simulink model "Copy_of_Clark"  (R2022b)
settings: Solver=ode4  StartTime=0.0  StopTime=1  FixedStep=1e-5  RelTol=1e-3
values from neighbouring files (symbols this model uses):
  E = 700    [FOCinit.m]
  f = 0.005    [FOCinit.m]
  J = 0.006    [FOCinit.m]
  Kie = 3 / (t5e * Ke)    (= 216000)    [FOCinit.m]
  Kif = 3 / (t5f * Kf)    (= 254.237288136)    [FOCinit.m]
  Kim = 3 / (t5m * Km)    (= 0.03)    [FOCinit.m]
  Kpe = taue * Kie    (= 2830.4)    [FOCinit.m]
  Kpf = tauf * Kif    (= 14.1242937853)    [FOCinit.m]
  Kpm = taum * Kim    (= 0.036)    [FOCinit.m]
  Lr = 0.075    [FOCinit.m]
  Ls = 0.280    (= 0.28)    [FOCinit.m]
  Msr = 0.118    [FOCinit.m]
  P = 2    [FOCinit.m]
  Poff = [1 1 1 1 1 1 1 1 1 1 1 1 1 1 1 1 1 1 ; 1 0 0 1 1 0 0 1 0 0 1 1 0 0 1 1 0 1; 1 1 0 0 1 0 0 1 1 0 0 1 1 0 1 1 0 0]'    [FOCinit.m]
  Rr = 1.35    [FOCinit.m]
  Rs = 7.2    [FOCinit.m]
  Ts = 1/fs    (= 0.0001)    [FOCinit.m]
libraries: slpidlib x4, simulink_extras x4, simulink x2, mcbcontrolslib x2
settings Model: Creator=ZinouAb  LastModifiedBy=ZinouAb
settings DebuggingCC: ParameterOverflowMsg=none  ParameterUnderflowMsg=error

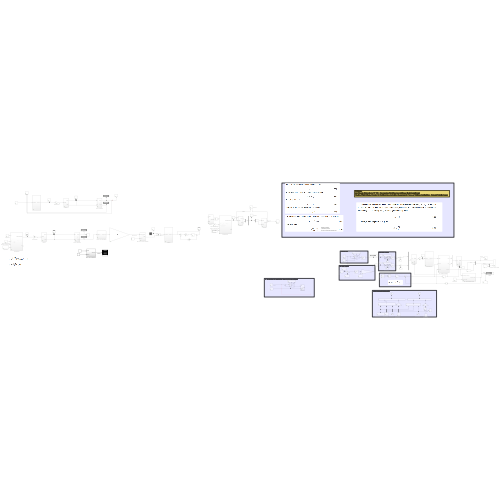
[thumbnail: Simulink's stored preview of the top-level diagram]
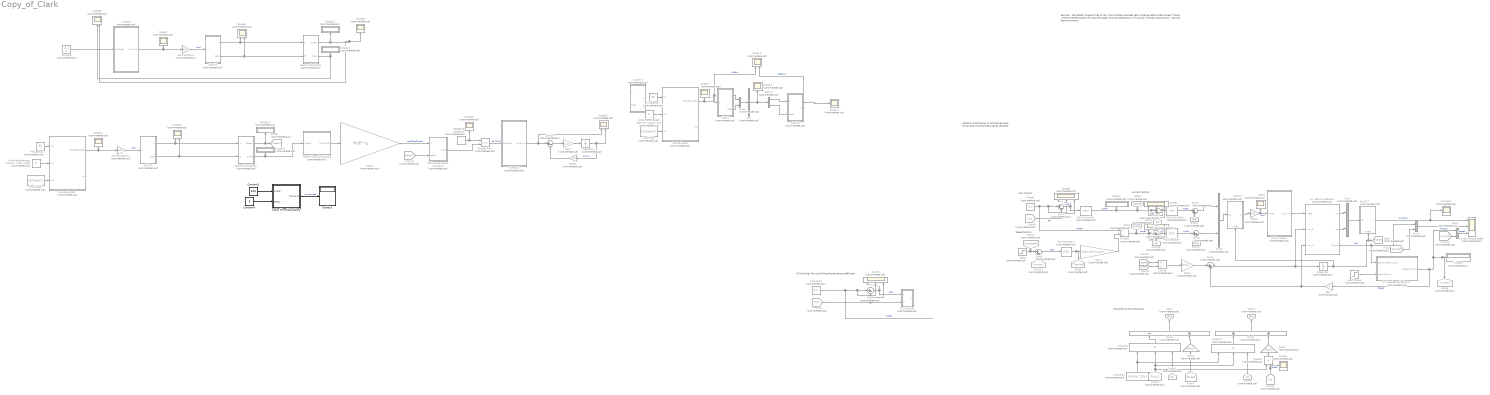
== system Copy_of_Clark ==
  note: Current Control
  note: Disturbance Compensation
  note: Notation Américaine:
      | p: Nombre de poles et
      | non pas le nombre des paires de poles
  note: Speed Control
  note: Sources :
      | Lab Sheets (Supports de TP UE - Commandes évoluées des systèmes électrotechniques)
      | Thesis : Field-Oriented Control for Squirrel-Cage Induction Generators in Pump as Turbines Applications - Samuel Ferreira Amaro
  note: Flux Control
  note: IP Controller (for controlling the damping coefficient)
  Alpha leDéphasage entre les courants (rad) : Constant  Commented=on  Value=0
  Alpha leDéphasage entre les courants (rad)1 : Constant  Commented=on  Value=0
  Amplitude : Constant  Commented=on  Value=220*sqrt(2)
  Amplitude1 : Constant  Commented=on  Value=220*sqrt(2)
  ClarkT : Subsystem  Commented=on
  ClarkT-1 : Subsystem  Commented=on
  ClarkT-2 : Subsystem  Commented=on
  ClarkT1 : Subsystem  Commented=on
  ClarkT2 : Subsystem  Commented=on
  Constant : Constant  Commented=on  Value=[1 1 0]
  Constant1 : Constant  Commented=on  Value=(Ls-(Msr^2)/Lr)
  Constant2 : Constant  Commented=on  Value=0.5
  Constant3 : Constant  Value=140
  Constant4 : Constant  Value=3
  CosineWaves : Subsystem  Commented=on
  CosineWaves1 : Subsystem  Commented=on
  Current,Torque,Speed : Scope  Commented=on  NumInputPorts=3
  Currents : Scope  Commented=on
  Demux : Demux  Commented=on  Outputs=2
  Display{,1..4} (5 alike) : Display  Commented=on
  Display5 : Display
  Divide : Product  Commented=on  Inputs=*/
  Divide1 : Product  Commented=on  Inputs=/*
  Frdref1 : Constant  Commented=on  Value=0.5
  From : From  Commented=on  GotoTag=Temref
  From1 : From  Commented=on  GotoTag=Isd  TagVisibility=global
  From10 : From  Commented=on  GotoTag=Frd  TagVisibility=global
  From11 : From  Commented=on  GotoTag=Isdref
  From12 : From  Commented=on  GotoTag=Isqref
  From13 : From  Commented=on  GotoTag=wmec
  From14 : From  Commented=on  GotoTag=wmecref
  From15 : From  Commented=on  GotoTag=Isq  TagVisibility=global
  From16 : From  Commented=on  GotoTag=Sector
  From2 : From  Commented=on  GotoTag=Ed
  From3 : From  Commented=on  GotoTag=Eq
  From4 : From  Commented=on  GotoTag=Puls_S  TagVisibility=global
  From5 : From  Commented=on  GotoTag=Isq  TagVisibility=global
  From6 : From  Commented=on  GotoTag=Frd  TagVisibility=global
  From7 : From  Commented=on  GotoTag=dFrddt  TagVisibility=global
  From8 : From  Commented=on  GotoTag=Isd  TagVisibility=global
  From9 : From  Commented=on  GotoTag=Frd  TagVisibility=global
  Fréquence : Constant  Commented=on  Value=50
  Fréquence1 : Constant  Commented=on  Value=50
  Gain : Gain  Commented=on  Gain=P
  Gain1 : Gain  Commented=on  Gain=(2/3)*(1/P)*(Lr/Msr)
  Gain2 : Gain  Commented=on  Gain=1/E
  Gain3 : Gain  Commented=on  Gain=Rr/Lr
  Gain4 : Gain  Commented=on  Gain=Msr/Lr
  Gain5 : Gain  Commented=on  Gain=Msr/Lr
  Gain6 : Gain  Commented=on  Gain=Poff  Multiplication=Matrix(K*u)
  Gain7 : Gain  Commented=on  Gain=1/Ls
  Gain8 : Gain  Commented=on  Gain=22
  Goto : Goto  Commented=on  GotoTag=Ed
  Goto1 : Goto  Commented=on  GotoTag=Eq
  Goto2 : Goto  Commented=on  GotoTag=Temref
  Goto3 : Goto  Commented=on  GotoTag=Isdref
  Goto4 : Goto  Commented=on  GotoTag=Isqref
  Goto5 : Goto  Commented=on  GotoTag=wmec
  Goto6 : Goto  Commented=on  GotoTag=wmecref
  Goto7 : Goto  Commented=on  GotoTag=thetas  TagVisibility=global
  Goto8 : Goto  Commented=on  GotoTag=Sector
  GreaterThan : RelationalOperator  Commented=on  OutDataTypeStr=boolean  RndMeth=Simplest  InputSameDT=off
  IM - Electric Behavior : Subsystem  Commented=on
  IM - Mechanical Behavior : Subsystem  Commented=on
  IP Controller : Subsystem  Commented=on
  Integrator : Integrator  Commented=on
  Integrator1 : Integrator  Commented=on
  Inverter : Subsystem  Commented=on
  Inverter1 : Subsystem  Commented=on
  Load Torque : Step  Commented=on  Time=2  After=0.5  SampleTime=0
  Mux : Mux  Commented=on  Inputs=1
  Mux{1..5} (5 alike) : Mux  Commented=on  Inputs=2
  "Normalization " : Gain  Commented=on  Gain=1/E
  Normalization 1 : Gain  Commented=on  Gain=1/E
  Off time per sector calculator : Subsystem  Commented=on
  PID Controller : slpidlib/PID Controller  Commented=on  Controller=PI  Form=Parallel  TimeDomain=Continuous-time  UseExternalTs=off  SampleTime=-1  IntegratorMethod=Forward Euler  FilterMethod=Forward Euler  ControllerParametersSource=internal  P=Kpe  I=Kie  UseKiTs=off  D=0  N=100  UseFilter=on  TunerSelectOption=Transfer Function Based (PID Tuner App)  InitialConditionSource=internal  InitialConditionForIntegrator=0  InitialConditionForFilter=0  DifferentiatorICPrevScaledInput=0  ExternalReset=none  TrackingMode=off  Kt=1  LimitOutput=off  SatLimitsSource=internal  UpperSaturationLimit=inf  LowerSaturationLimit=-inf  LinearizeAsGain=on  AntiWindupMode=none  Kb=1  LimitIntegrator=off  UpperIntegratorSaturationLimit=inf  LowerIntegratorSaturationLimit=-inf  POutMin=[]  POutMax=[]  IOutMin=[]  IOutMax=[]  DOutMin=[]  DOutMax=[]  NOutMin=[]  NOutMax=[]  SumOutMin=[]  SumOutMax=[]  SaturationOutMin=[]  SaturationOutMax=[]  PParamMin=[]  PParamMax=[]  IParamMin=[]  IParamMax=[]  DParamMin=[]  DParamMax=[]  NParamMin=[]  NParamMax=[]  KbParamMin=[]  KbParamMax=[]  KtParamMin=[]  KtParamMax=[]  KbOutMin=[]  KbOutMax=[]  KtOutMin=[]  KtOutMax=[]  IntegratorOutMin=[]  IntegratorOutMax=[]  FilterOutMin=[]  FilterOutMax=[]  SumI1OutMin=[]  SumI1OutMax=[]  SumI2OutMin=[]  SumI2OutMax=[]  SumI3OutMin=[]  SumI3OutMax=[]  SumI4OutMin=[]  SumI4OutMax=[]  SumDOutMin=[]  SumDOutMax=[]  DifferentiatorOutMin=[]  DifferentiatorOutMax=[]  FilterDiffOutCoefMin=[]  FilterDiffOutCoefMax=[]  ReciprocalOutMin=[]  ReciprocalOutMax=[]  SumDenOutMin=[]  SumDenOutMax=[]  SumNumOutMin=[]  SumNumOutMax=[]  DivideOutMin=[]  DivideOutMax=[]  UdiffTsProdOutMin=[]  UdiffTsProdOutMax=[]  NTsProdOutMin=[]  NTsProdOutMax=[]  UintegralTsProdOutMin=[]  UintegralTsProdOutMax=[]  UngainTsProdOutMin=[]  UngainTsProdOutMax=[]  ClampingZeroOutDataTypeStr=Inherit: Inherit via back propagation  ClampingZeroOutMin=[]  ClampingZeroOutMax=[]  FilterDenConstantOutDataTypeStr=Inherit: Inherit via back propagation  FilterDenConstantOutMin=[]  FilterDenConstantOutMax=[]  PCopyOutDataTypeStr=Inherit: Inherit via back propagation  PCopyOutMin=[]  PCopyOutMax=[]  NCopyOutDataTypeStr=Inherit: Inherit via back propagation  NCopyOutMin=[]  NCopyOutMax=[]  IntegratorContinuousStateAttributes=''  IntegratorStateMustResolveToSignalObject=off  IntegratorRTWStateStorageClass=Auto  FilterContinuousStateAttributes=''  FilterStateMustResolveToSignalObject=off  FilterRTWStateStorageClass=Auto  ParallelPVariant=InternalParameters  IdealPVariant=Disabled  IVariant=InternalParameters  DVariant=Disabled  IntegratorVariant=Continuous  SatVariant=Disabled  AWVariant=Passthrough  PCopyVariant=Disabled  TRVariant=Disabled  FdbkBlocksVariant=Forward  IdealPFdbkVariant=Disabled  SatFdbkVariant=Disabled  DerivativeFilterVariant=Disabled  NVariant=Disabled  NCopyVariant=Disabled_SignalSpec  FilterICVariant=Disabled  IntegratorICVariant=InternalICs  ExternalResetVariant=Disabled  TRSumVariant=Passthrough  SumFdbkVariant=Disabled  SumVariant=Sum_PI  TsampFilterVariant=InternalTs  TsampNgainVariant=Passthrough  TsampIntegralVariant=Passthrough  ExternalSaturationOutDataTypeStr=Inherit: Same as second input
  PID Controller1 : slpidlib/PID Controller  Commented=on  Controller=PI  Form=Parallel  TimeDomain=Continuous-time  UseExternalTs=off  SampleTime=-1  IntegratorMethod=Forward Euler  FilterMethod=Forward Euler  ControllerParametersSource=internal  P=Kpe  I=Kie  UseKiTs=off  D=0  N=100  UseFilter=on  TunerSelectOption=Transfer Function Based (PID Tuner App)  InitialConditionSource=internal  InitialConditionForIntegrator=0  InitialConditionForFilter=0  DifferentiatorICPrevScaledInput=0  ExternalReset=none  TrackingMode=off  Kt=1  LimitOutput=off  SatLimitsSource=internal  UpperSaturationLimit=inf  LowerSaturationLimit=-inf  LinearizeAsGain=on  AntiWindupMode=none  Kb=1  LimitIntegrator=off  UpperIntegratorSaturationLimit=inf  LowerIntegratorSaturationLimit=-inf  POutMin=[]  POutMax=[]  IOutMin=[]  IOutMax=[]  DOutMin=[]  DOutMax=[]  NOutMin=[]  NOutMax=[]  SumOutMin=[]  SumOutMax=[]  SaturationOutMin=[]  SaturationOutMax=[]  PParamMin=[]  PParamMax=[]  IParamMin=[]  IParamMax=[]  DParamMin=[]  DParamMax=[]  NParamMin=[]  NParamMax=[]  KbParamMin=[]  KbParamMax=[]  KtParamMin=[]  KtParamMax=[]  KbOutMin=[]  KbOutMax=[]  KtOutMin=[]  KtOutMax=[]  IntegratorOutMin=[]  IntegratorOutMax=[]  FilterOutMin=[]  FilterOutMax=[]  SumI1OutMin=[]  SumI1OutMax=[]  SumI2OutMin=[]  SumI2OutMax=[]  SumI3OutMin=[]  SumI3OutMax=[]  SumI4OutMin=[]  SumI4OutMax=[]  SumDOutMin=[]  SumDOutMax=[]  DifferentiatorOutMin=[]  DifferentiatorOutMax=[]  FilterDiffOutCoefMin=[]  FilterDiffOutCoefMax=[]  ReciprocalOutMin=[]  ReciprocalOutMax=[]  SumDenOutMin=[]  SumDenOutMax=[]  SumNumOutMin=[]  SumNumOutMax=[]  DivideOutMin=[]  DivideOutMax=[]  UdiffTsProdOutMin=[]  UdiffTsProdOutMax=[]  NTsProdOutMin=[]  NTsProdOutMax=[]  UintegralTsProdOutMin=[]  UintegralTsProdOutMax=[]  UngainTsProdOutMin=[]  UngainTsProdOutMax=[]  ClampingZeroOutDataTypeStr=Inherit: Inherit via back propagation  ClampingZeroOutMin=[]  ClampingZeroOutMax=[]  FilterDenConstantOutDataTypeStr=Inherit: Inherit via back propagation  FilterDenConstantOutMin=[]  FilterDenConstantOutMax=[]  PCopyOutDataTypeStr=Inherit: Inherit via back propagation  PCopyOutMin=[]  PCopyOutMax=[]  NCopyOutDataTypeStr=Inherit: Inherit via back propagation  NCopyOutMin=[]  NCopyOutMax=[]  IntegratorContinuousStateAttributes=''  IntegratorStateMustResolveToSignalObject=off  IntegratorRTWStateStorageClass=Auto  FilterContinuousStateAttributes=''  FilterStateMustResolveToSignalObject=off  FilterRTWStateStorageClass=Auto  ParallelPVariant=InternalParameters  IdealPVariant=Disabled  IVariant=InternalParameters  DVariant=Disabled  IntegratorVariant=Continuous  SatVariant=Disabled  AWVariant=Passthrough  PCopyVariant=Disabled  TRVariant=Disabled  FdbkBlocksVariant=Forward  IdealPFdbkVariant=Disabled  SatFdbkVariant=Disabled  DerivativeFilterVariant=Disabled  NVariant=Disabled  NCopyVariant=Disabled_SignalSpec  FilterICVariant=Disabled  IntegratorICVariant=InternalICs  ExternalResetVariant=Disabled  TRSumVariant=Passthrough  SumFdbkVariant=Disabled  SumVariant=Sum_PI  TsampFilterVariant=InternalTs  TsampNgainVariant=Passthrough  TsampIntegralVariant=Passthrough  ExternalSaturationOutDataTypeStr=Inherit: Same as second input
  PID Controller2 : slpidlib/PID Controller  Commented=on  Controller=PI  Form=Parallel  TimeDomain=Continuous-time  UseExternalTs=off  SampleTime=-1  IntegratorMethod=Forward Euler  FilterMethod=Forward Euler  ControllerParametersSource=internal  P=Kpf  I=Kif  UseKiTs=off  D=0  N=100  UseFilter=on  TunerSelectOption=Transfer Function Based (PID Tuner App)  InitialConditionSource=internal  InitialConditionForIntegrator=0  InitialConditionForFilter=0  DifferentiatorICPrevScaledInput=0  ExternalReset=none  TrackingMode=off  Kt=1  LimitOutput=off  SatLimitsSource=internal  UpperSaturationLimit=inf  LowerSaturationLimit=-inf  LinearizeAsGain=on  AntiWindupMode=none  Kb=1  LimitIntegrator=off  UpperIntegratorSaturationLimit=inf  LowerIntegratorSaturationLimit=-inf  POutMin=[]  POutMax=[]  IOutMin=[]  IOutMax=[]  DOutMin=[]  DOutMax=[]  NOutMin=[]  NOutMax=[]  SumOutMin=[]  SumOutMax=[]  SaturationOutMin=[]  SaturationOutMax=[]  PParamMin=[]  PParamMax=[]  IParamMin=[]  IParamMax=[]  DParamMin=[]  DParamMax=[]  NParamMin=[]  NParamMax=[]  KbParamMin=[]  KbParamMax=[]  KtParamMin=[]  KtParamMax=[]  KbOutMin=[]  KbOutMax=[]  KtOutMin=[]  KtOutMax=[]  IntegratorOutMin=[]  IntegratorOutMax=[]  FilterOutMin=[]  FilterOutMax=[]  SumI1OutMin=[]  SumI1OutMax=[]  SumI2OutMin=[]  SumI2OutMax=[]  SumI3OutMin=[]  SumI3OutMax=[]  SumI4OutMin=[]  SumI4OutMax=[]  SumDOutMin=[]  SumDOutMax=[]  DifferentiatorOutMin=[]  DifferentiatorOutMax=[]  FilterDiffOutCoefMin=[]  FilterDiffOutCoefMax=[]  ReciprocalOutMin=[]  ReciprocalOutMax=[]  SumDenOutMin=[]  SumDenOutMax=[]  SumNumOutMin=[]  SumNumOutMax=[]  DivideOutMin=[]  DivideOutMax=[]  UdiffTsProdOutMin=[]  UdiffTsProdOutMax=[]  NTsProdOutMin=[]  NTsProdOutMax=[]  UintegralTsProdOutMin=[]  UintegralTsProdOutMax=[]  UngainTsProdOutMin=[]  UngainTsProdOutMax=[]  ClampingZeroOutDataTypeStr=Inherit: Inherit via back propagation  ClampingZeroOutMin=[]  ClampingZeroOutMax=[]  FilterDenConstantOutDataTypeStr=Inherit: Inherit via back propagation  FilterDenConstantOutMin=[]  FilterDenConstantOutMax=[]  PCopyOutDataTypeStr=Inherit: Inherit via back propagation  PCopyOutMin=[]  PCopyOutMax=[]  NCopyOutDataTypeStr=Inherit: Inherit via back propagation  NCopyOutMin=[]  NCopyOutMax=[]  IntegratorContinuousStateAttributes=''  IntegratorStateMustResolveToSignalObject=off  IntegratorRTWStateStorageClass=Auto  FilterContinuousStateAttributes=''  FilterStateMustResolveToSignalObject=off  FilterRTWStateStorageClass=Auto  ParallelPVariant=InternalParameters  IdealPVariant=Disabled  IVariant=InternalParameters  DVariant=Disabled  IntegratorVariant=Continuous  SatVariant=Disabled  AWVariant=Passthrough  PCopyVariant=Disabled  TRVariant=Disabled  FdbkBlocksVariant=Forward  IdealPFdbkVariant=Disabled  SatFdbkVariant=Disabled  DerivativeFilterVariant=Disabled  NVariant=Disabled  NCopyVariant=Disabled_SignalSpec  FilterICVariant=Disabled  IntegratorICVariant=InternalICs  ExternalResetVariant=Disabled  TRSumVariant=Passthrough  SumFdbkVariant=Disabled  SumVariant=Sum_PI  TsampFilterVariant=InternalTs  TsampNgainVariant=Passthrough  TsampIntegralVariant=Passthrough  ExternalSaturationOutDataTypeStr=Inherit: Same as second input
  PID Controller3 : slpidlib/PID Controller  Commented=on  Controller=PI  Form=Parallel  TimeDomain=Continuous-time  UseExternalTs=off  SampleTime=-1  IntegratorMethod=Forward Euler  FilterMethod=Forward Euler  ControllerParametersSource=internal  P=Kpm  I=Kim  UseKiTs=off  D=0  N=100  UseFilter=on  TunerSelectOption=Transfer Function Based (PID Tuner App)  InitialConditionSource=internal  InitialConditionForIntegrator=0  InitialConditionForFilter=0  DifferentiatorICPrevScaledInput=0  ExternalReset=none  TrackingMode=off  Kt=1  LimitOutput=off  SatLimitsSource=internal  UpperSaturationLimit=inf  LowerSaturationLimit=-inf  LinearizeAsGain=on  AntiWindupMode=none  Kb=1  LimitIntegrator=off  UpperIntegratorSaturationLimit=inf  LowerIntegratorSaturationLimit=-inf  POutMin=[]  POutMax=[]  IOutMin=[]  IOutMax=[]  DOutMin=[]  DOutMax=[]  NOutMin=[]  NOutMax=[]  SumOutMin=[]  SumOutMax=[]  SaturationOutMin=[]  SaturationOutMax=[]  PParamMin=[]  PParamMax=[]  IParamMin=[]  IParamMax=[]  DParamMin=[]  DParamMax=[]  NParamMin=[]  NParamMax=[]  KbParamMin=[]  KbParamMax=[]  KtParamMin=[]  KtParamMax=[]  KbOutMin=[]  KbOutMax=[]  KtOutMin=[]  KtOutMax=[]  IntegratorOutMin=[]  IntegratorOutMax=[]  FilterOutMin=[]  FilterOutMax=[]  SumI1OutMin=[]  SumI1OutMax=[]  SumI2OutMin=[]  SumI2OutMax=[]  SumI3OutMin=[]  SumI3OutMax=[]  SumI4OutMin=[]  SumI4OutMax=[]  SumDOutMin=[]  SumDOutMax=[]  DifferentiatorOutMin=[]  DifferentiatorOutMax=[]  FilterDiffOutCoefMin=[]  FilterDiffOutCoefMax=[]  ReciprocalOutMin=[]  ReciprocalOutMax=[]  SumDenOutMin=[]  SumDenOutMax=[]  SumNumOutMin=[]  SumNumOutMax=[]  DivideOutMin=[]  DivideOutMax=[]  UdiffTsProdOutMin=[]  UdiffTsProdOutMax=[]  NTsProdOutMin=[]  NTsProdOutMax=[]  UintegralTsProdOutMin=[]  UintegralTsProdOutMax=[]  UngainTsProdOutMin=[]  UngainTsProdOutMax=[]  ClampingZeroOutDataTypeStr=Inherit: Inherit via back propagation  ClampingZeroOutMin=[]  ClampingZeroOutMax=[]  FilterDenConstantOutDataTypeStr=Inherit: Inherit via back propagation  FilterDenConstantOutMin=[]  FilterDenConstantOutMax=[]  PCopyOutDataTypeStr=Inherit: Inherit via back propagation  PCopyOutMin=[]  PCopyOutMax=[]  NCopyOutDataTypeStr=Inherit: Inherit via back propagation  NCopyOutMin=[]  NCopyOutMax=[]  IntegratorContinuousStateAttributes=''  IntegratorStateMustResolveToSignalObject=off  IntegratorRTWStateStorageClass=Auto  FilterContinuousStateAttributes=''  FilterStateMustResolveToSignalObject=off  FilterRTWStateStorageClass=Auto  ParallelPVariant=InternalParameters  IdealPVariant=Disabled  IVariant=InternalParameters  DVariant=Disabled  IntegratorVariant=Continuous  SatVariant=Disabled  AWVariant=Passthrough  PCopyVariant=Disabled  TRVariant=Disabled  FdbkBlocksVariant=Forward  IdealPFdbkVariant=Disabled  SatFdbkVariant=Disabled  DerivativeFilterVariant=Disabled  NVariant=Disabled  NCopyVariant=Disabled_SignalSpec  FilterICVariant=Disabled  IntegratorICVariant=InternalICs  ExternalResetVariant=Disabled  TRSumVariant=Passthrough  SumFdbkVariant=Disabled  SumVariant=Sum_PI  TsampFilterVariant=InternalTs  TsampNgainVariant=Passthrough  TsampIntegralVariant=Passthrough  ExternalSaturationOutDataTypeStr=Inherit: Same as second input
  PWM Inverter : Subsystem  Commented=on
  ParkT-2 : Subsystem  Commented=on
      settings: PortSchema="{\"entries\":[{\"content\":{\"sides\":[{\"content\":{\"connectorIds\":[\"In1\"]},\"type\":\"ConnectorPlacement.EquallySpacedRectSide\",\"uuid\":\"ed5ee07b-b316-480c-b9ec-652acf4aaee1\"},{\"content\":{\"connectorIds\":[\"Out1\"],\"side\":\"RIGHT\"},\"type\":\"ConnectorPlacement.EquallySpacedRectSide\",\"uuid\":\"52d50e66-916b-4a4a-9cee-3d7b4015ccc4\"},{\"content\":{\"connectorIds\":[],\"side\":\"TOP\"},\"type\":\"ConnectorPlacement.EquallySpacedRectSide\",\"uuid\":\"08f86e0e-d4d6-4b18-9159-89a705b15501\"},{\"content\":{\"connectorIds\":[\"In2\"],\"side\":\"BOTTOM\"},\"type\":\"ConnectorPlacement.EquallySpacedRectSide\",\"uuid\":\"c8ae1c02-6dab-4f60-b9b6-1b5db27b47ec\"}]},\"type\":\"ConnectorPlacement.EquallySpacedConnector\",\"uuid\":\"6fabca93-26c3-4fea-833e-475510973df7\"}],\"packageUris\":[\"http://schema.mathworks.com/mf0/Connector/R2020b\"],\"version\":\"1.0\"}"
  ParkT-3 : Subsystem  Commented=on
      settings: PortSchema="{\"entries\":[{\"content\":{\"sides\":[{\"content\":{\"connectorIds\":[\"In1\"]},\"type\":\"ConnectorPlacement.EquallySpacedRectSide\",\"uuid\":\"ed5ee07b-b316-480c-b9ec-652acf4aaee1\"},{\"content\":{\"connectorIds\":[\"Out1\"],\"side\":\"RIGHT\"},\"type\":\"ConnectorPlacement.EquallySpacedRectSide\",\"uuid\":\"52d50e66-916b-4a4a-9cee-3d7b4015ccc4\"},{\"content\":{\"connectorIds\":[],\"side\":\"TOP\"},\"type\":\"ConnectorPlacement.EquallySpacedRectSide\",\"uuid\":\"08f86e0e-d4d6-4b18-9159-89a705b15501\"},{\"content\":{\"connectorIds\":[\"In2\"],\"side\":\"BOTTOM\"},\"type\":\"ConnectorPlacement.EquallySpacedRectSide\",\"uuid\":\"c8ae1c02-6dab-4f60-b9b6-1b5db27b47ec\"}]},\"type\":\"ConnectorPlacement.EquallySpacedConnector\",\"uuid\":\"6fabca93-26c3-4fea-833e-475510973df7\"}],\"packageUris\":[\"http://schema.mathworks.com/mf0/Connector/R2020b\"],\"version\":\"1.0\"}"
  Product : Product  Commented=on
  Product1 : Product  Commented=on  Inputs=3
  Product2 : Product  Commented=on  Inputs=3
  Repeating Sequence : simulink/Sources/Repeating Sequence  Commented=on  rep_seq_t=[0 Ts 2*Ts]  rep_seq_y=[0 1 0]
  Scope{,2,7..8,11,13} (6 alike) : Scope  Commented=on
  Scope 1 : Scope  Commented=on
  Scope 2 : Scope  Commented=on
  Scope 3 : Scope  Commented=on  NumInputPorts=2
  Scope 4 : Scope  Commented=on
  Scope{1,3..5,9} (5 alike) : Scope  Commented=on  NumInputPorts=3
  Scope10 : Scope  Commented=on  NumInputPorts=2
  Scope12 : Scope  Commented=on  NumInputPorts=2
  Scope6 : Scope  Commented=on  NumInputPorts=2
  Sector Calculation : Subsystem  Commented=on
  Sector Calculation1 : Subsystem  Commented=on
  Step1 : Step  Commented=on  After=150  SampleTime=0
  Sum{,1,7..10} (6 alike) : Sum  Commented=on  Inputs=|+-
  Sum2 : Sum  Commented=on  Inputs=|++
  Sum3 : Sum  Commented=on  Inputs=|++
  Sum4 : Sum  Commented=on  Inputs=|++
  Sum5 : Sum  Commented=on  Inputs=-+
  Sum6 : Sum  Commented=on
  Vactor Time Calculation1 : Subsystem
  Vactor Time Calculation2 : Subsystem  Commented=on
  Vitesse : Display  Commented=on
  wires:
  Mux1/1 -> Mux/1
  Mux/1 -> Demux/1, Scope 2/1
  ClarkT-1/1(XABC) -> Scope 3/2, Scope 4/1  "XABCout"
  Amplitude/1 -> CosineWaves/3(In3)
  Alpha leDéphasage entre les courants (rad)/1 -> CosineWaves/2(In2)
  Fréquence/1 -> CosineWaves/1(In1)
  CosineWaves/1(COSINEWAVES) -> ClarkT/1(XABC), Scope 3/1, Scope 1/1  "XABCin"
  ClarkT/1(alpha) -> Mux1/1
  ClarkT/2(beta) -> Mux1/2
  Demux/1 -> ClarkT-1/1(alpha)
  Demux/2 -> ClarkT-1/2(beta)
  Mux3/1 -> Current,Torque,Speed/3  "Speed"
  ParkT-3/1(XABC) -> Currents/1, Current,Torque,Speed/1  "Currents"
  Step1/1 -> Sum9/1, Goto6/1
  ParkT-2/1(XABC) -> Gain2/1
  Mux5/1 -> ParkT-2/1(dq)
  From11/1 -> Divide/2
  Product2/1 -> Sum5/1
  From6/1 -> Scope2/1, Product/2  "Frdref"
  Product/1 -> Gain5/1
  PID Controller3/1 -> Goto2/1, Gain1/1
  Gain5/1 -> Sum6/2
  Mux2/1 -> Current,Torque,Speed/2  "Torque"
  Sum/1 -> Scope5/1, PID Controller/1  "diffq"
  From1/1 -> Scope1/3, Sum1/2  "Isd"
  Gain1/1 -> Divide1/2
  From15/1 -> Scope5/3, Sum/2  "Isq"
  From7/1 -> Gain4/1
  Product1/1 -> Sum6/1
  Sum4/1 -> IM - Electric Behavior/2(Puls_S), Integrator/1
  Integrator/1 -> ParkT-2/2(Theta), ParkT-3/2(Theta), Goto7/1
  Gain3/1 -> Sum4/1
  Divide/1 -> Gain3/1
  Load Torque/1 -> IM - Mechanical Behavior/2(Load Torque)
  Sum9/1 -> PID Controller3/1  "Diff"
  From3/1 -> Sum2/2
  From2/1 -> Sum3/2
  From/1 -> Mux2/2
  Mux4/1 -> ParkT-3/1(dq)
  Sum2/1 -> Mux5/2
  Sum1/1 -> PID Controller1/1, Scope1/1  "diffd"
  IM - Mechanical Behavior/1(Speed (rad/s)) -> Mux3/1, Goto5/1, Vitesse/1, Gain/1  "Speed"
  Sum3/1 -> Mux5/1
  Gain/1 -> Sum4/2, IM - Electric Behavior/3(Puls_M)
  PID Controller1/1 -> Sum3/1  "Vd-Ed"
  IM - Electric Behavior/1(Isd) -> Mux4/1
  IM - Electric Behavior/2(Isq) -> Mux4/2
  Frdref1/1 -> Divide1/1, Scope3/2, Sum7/1  "Frdref"
  PWM Inverter/1(Va,Vb,Vc) -> IM - Electric Behavior/1(VABC)
  From9/1 -> Scope3/3, Sum7/2  "Frd"
  PID Controller2/1 -> Goto3/1, Scope1/2, Sum1/1, Display/1  "Isdref"
  From4/1 -> Product1/2, Product2/2, Product/1
  Constant2/1 -> Scope4/2, Sum8/1  "Frdref"
  Constant1/1 -> Product2/1, Product1/1
  PID Controller/1 -> Sum2/1  "Vq-Eq"
  Sum6/1 -> Goto1/1
  Sum5/1 -> Goto/1
  From10/1 -> IP Controller/2(meas), Scope4/3, Sum8/2
  Gain4/1 -> Sum5/2
  IM - Electric Behavior/3(Torque) -> Mux2/1, IM - Mechanical Behavior/1(Developed Torque)  "Tem"
  From14/1 -> Mux3/2
  From5/1 -> Product2/3
  From12/1 -> Divide/1
  Divide1/1 -> Goto4/1, Scope5/2, Sum/1  "Isqref"
  Sum8/1 -> IP Controller/1(Diff), Scope4/1  "Diff"
  Sum7/1 -> PID Controller2/1, Scope3/1  "Diff"
  From13/1 -> Sum9/2
  From8/1 -> Product1/3
  Gain2/1 -> Scope/1, PWM Inverter/1(mABX)  "Mod"
  "Normalization "/1 -> ClarkT1/1(XABC)  "Mod"
  Inverter/1(Va,Vb,Vc) -> Scope7/1, "Normalization "/1
  ClarkT1/1(alpha) -> Scope6/1, Sector Calculation/1(A)
  ClarkT1/2(beta) -> Scope6/2, Sector Calculation/2(B)
  Sector Calculation/1(Sector) -> Scope8/1, Scope9/3, Display1/1
  Sector Calculation/2(Angle) -> Scope9/2, Display2/1
  Constant/1 -> Inverter/1(Ca,Cb,Cc)
  Sector Calculation1/2(Angle) -> Vactor Time Calculation2/1(Angle°), Display4/1
  Sector Calculation1/1(Sector) -> Goto8/1, Display3/1
  ClarkT2/2(beta) -> Sector Calculation1/2(B), Scope10/2
  ClarkT2/1(alpha) -> Sector Calculation1/1(A), Scope10/1
  CosineWaves1/1(COSINEWAVES) -> Normalization 1/1, Scope11/1
  Normalization 1/1 -> ClarkT2/1(XABC)  "Mod"
  Vactor Time Calculation2/1(T0/2,t1,t2) -> Gain6/1
  Repeating Sequence/1 -> Scope13/1, GreaterThan/1
  GreaterThan/1 -> Inverter1/1(Ca,Cb,Cc)  "Ca,Cb,Cc"
  Gain6/1 -> Off time per sector calculator/1(taoff,tboff,tcoff)  "taoff,tboff,tcoff"
  From16/1 -> Off time per sector calculator/2(sector)
  Off time per sector calculator/1(Tmat) -> GreaterThan/2
  Fréquence1/1 -> CosineWaves1/1(In1)
  Amplitude1/1 -> CosineWaves1/3(In3)
  Alpha leDéphasage entre les courants (rad)1/1 -> CosineWaves1/2(In2)
  Inverter1/1(Va,Vb,Vc) -> Scope12/1, Sum10/1
  Sum10/1 -> Gain7/1
  Gain8/1 -> Sum10/2
  Gain7/1 -> Integrator1/1
  Integrator1/1 -> Scope12/2, Gain8/1  "Ia,Ib,Ic"
  Constant3/1 -> Vactor Time Calculation1/1(Angle°)
  Vactor Time Calculation1/1(T0/2,t1,t2) -> Display5/1  "normalized"
  Constant4/1 -> Vactor Time Calculation1/2(Sector)

== system Copy_of_Clark/ClarkT ==
  XABC : Inport
  MATLAB Function1 : MATLAB Function  TreatAsAtomicUnit=on
  alpha : Outport
  beta : Outport  Port=2
  wires:
  MATLAB Function1/1(alpha) -> alpha/1
  XABC/1 -> MATLAB Function1/1(x)
  MATLAB Function1/2(beta) -> beta/1

== system Copy_of_Clark/ClarkT-1 ==
  alpha : Inport
  beta : Inport  Port=2
  MATLAB Function : MATLAB Function  TreatAsAtomicUnit=on
  XABC : Outport
  wires:
  MATLAB Function/1(XABC) -> XABC/1
  alpha/1 -> MATLAB Function/1(alpha)
  beta/1 -> MATLAB Function/2(beta)

== system Copy_of_Clark/ClarkT-2 ==
  alpha : Inport
  beta : Inport  Port=2
  MATLAB Function : MATLAB Function  TreatAsAtomicUnit=on
  XABC : Outport
  wires:
  MATLAB Function/1(XABC) -> XABC/1
  alpha/1 -> MATLAB Function/1(alpha)
  beta/1 -> MATLAB Function/2(beta)

== system Copy_of_Clark/ClarkT1 ==
  XABC : Inport
  MATLAB Function1 : MATLAB Function  TreatAsAtomicUnit=on
  alpha : Outport
  beta : Outport  Port=2
  wires:
  MATLAB Function1/1(alpha) -> alpha/1
  XABC/1 -> MATLAB Function1/1(x)
  MATLAB Function1/2(beta) -> beta/1

== system Copy_of_Clark/ClarkT2 ==
  XABC : Inport
  MATLAB Function1 : MATLAB Function  TreatAsAtomicUnit=on
  alpha : Outport
  beta : Outport  Port=2
  wires:
  MATLAB Function1/2(beta) -> beta/1
  XABC/1 -> MATLAB Function1/1(x)
  MATLAB Function1/1(alpha) -> alpha/1

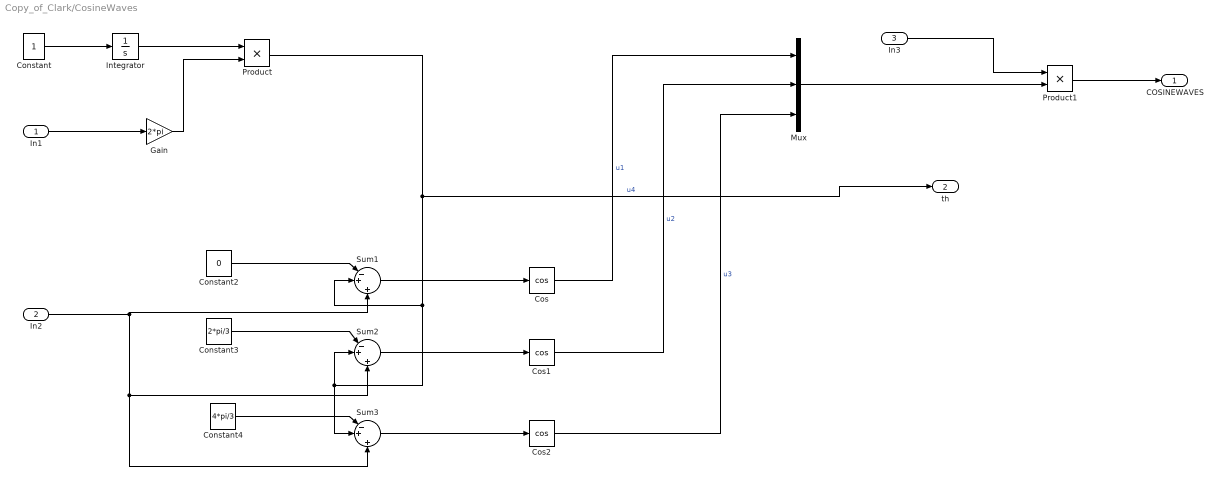
== system Copy_of_Clark/CosineWaves ==
  In1 : Inport
  In2 : Inport  Port=2
  In3 : Inport  Port=3
  Constant : Constant
  Constant2 : Constant  Value=0
  Constant3 : Constant  Value=2*pi/3
  Constant4 : Constant  Value=4*pi/3
  Cos : Trigonometry  Operator=cos
  Cos1 : Trigonometry  Operator=cos
  Cos2 : Trigonometry  Operator=cos
  Gain : Gain  Gain=2*pi
  Integrator : Integrator
  Mux : Mux  Inputs=3
  Product : Product
  Product1 : Product
  Sum1 : Sum  Inputs=|-+|+
  Sum2 : Sum  Inputs=|-+|+
  Sum3 : Sum  Inputs=|-+|+
  COSINEWAVES : Outport
  th : Outport  Port=2
  wires:
  Constant/1 -> Integrator/1
  Sum2/1 -> Cos1/1
  In2/1 -> Sum1/3, Sum3/3, Sum2/3
  Product/1 -> th/1, Sum3/2, Sum2/2, Sum1/2  "u4"
  Constant3/1 -> Sum2/1
  Sum3/1 -> Cos2/1
  Sum1/1 -> Cos/1
  Constant2/1 -> Sum1/1
  Constant4/1 -> Sum3/1
  Gain/1 -> Product/2
  Integrator/1 -> Product/1
  In1/1 -> Gain/1
  Cos1/1 -> Mux/2  "u2"
  Cos/1 -> Mux/1  "u1"
  Cos2/1 -> Mux/3  "u3"
  Mux/1 -> Product1/2
  In3/1 -> Product1/1
  Product1/1 -> COSINEWAVES/1

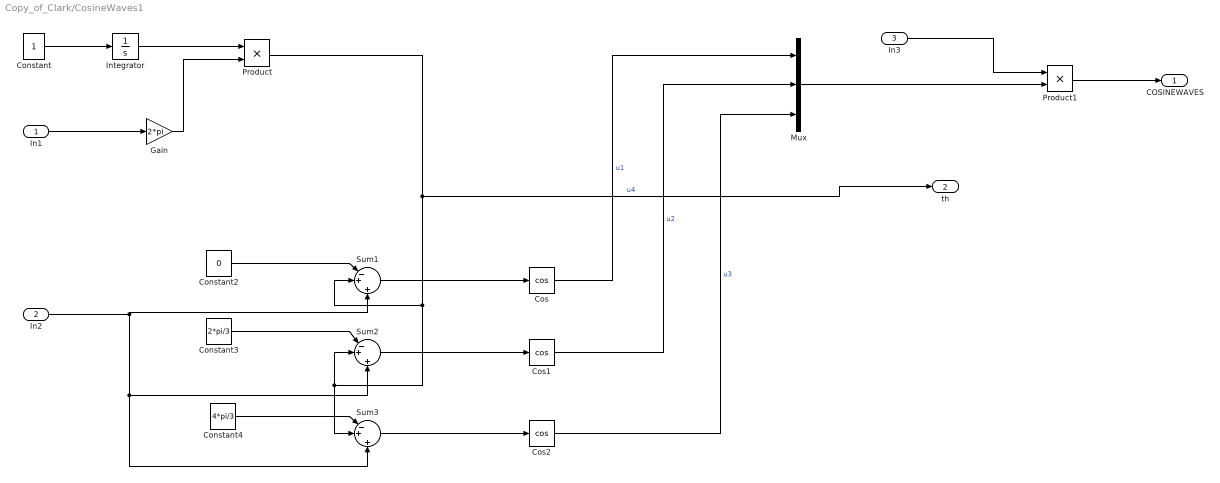
== system Copy_of_Clark/CosineWaves1 ==
  In1 : Inport
  In2 : Inport  Port=2
  In3 : Inport  Port=3
  Constant : Constant
  Constant2 : Constant  Value=0
  Constant3 : Constant  Value=2*pi/3
  Constant4 : Constant  Value=4*pi/3
  Cos : Trigonometry  Operator=cos
  Cos1 : Trigonometry  Operator=cos
  Cos2 : Trigonometry  Operator=cos
  Gain : Gain  Gain=2*pi
  Integrator : Integrator
  Mux : Mux  Inputs=3
  Product : Product
  Product1 : Product
  Sum1 : Sum  Inputs=|-+|+
  Sum2 : Sum  Inputs=|-+|+
  Sum3 : Sum  Inputs=|-+|+
  COSINEWAVES : Outport
  th : Outport  Port=2
  wires:
  Constant/1 -> Integrator/1
  Sum2/1 -> Cos1/1
  In2/1 -> Sum1/3, Sum3/3, Sum2/3
  Product/1 -> th/1, Sum3/2, Sum2/2, Sum1/2  "u4"
  Constant3/1 -> Sum2/1
  Sum3/1 -> Cos2/1
  Sum1/1 -> Cos/1
  Constant2/1 -> Sum1/1
  Constant4/1 -> Sum3/1
  Gain/1 -> Product/2
  Integrator/1 -> Product/1
  In1/1 -> Gain/1
  Cos1/1 -> Mux/2  "u2"
  Cos/1 -> Mux/1  "u1"
  Cos2/1 -> Mux/3  "u3"
  Mux/1 -> Product1/2
  In3/1 -> Product1/1
  Product1/1 -> COSINEWAVES/1

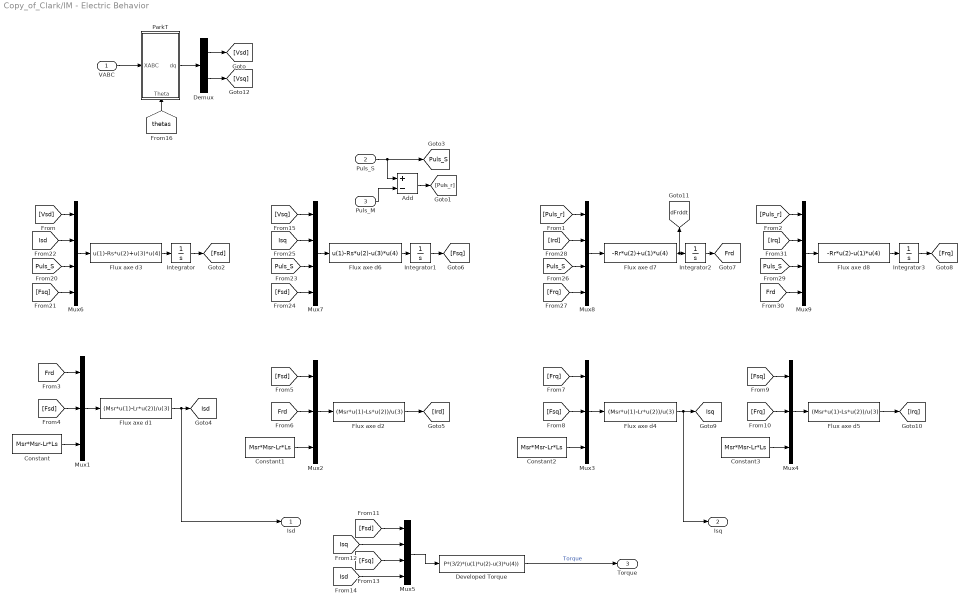
== system Copy_of_Clark/IM - Electric Behavior ==
  VABC : Inport
  Puls_S : Inport  Port=2
  Puls_M : Inport  Port=3
  Add : Sum  Inputs=+-
  Constant{,1..3} (4 alike) : Constant  Value=Msr*Msr-Lr*Ls
  Demux : Demux  Outputs=2
  Developed Torque : Fcn  Expr=P*(3/2)*(u(1)*u(2)-u(3)*u(4))
  Flux axe d1 : Fcn  Expr=(Msr*u(1)-Lr*u(2))/u(3)
  Flux axe d2 : Fcn  Expr=(Msr*u(1)-Ls*u(2))/u(3)
  Flux axe d3 : Fcn  Expr=u(1)-Rs*u(2)+u(3)*u(4)
  Flux axe d4 : Fcn  Expr=(Msr*u(1)-Lr*u(2))/u(3)
  Flux axe d5 : Fcn  Expr=(Msr*u(1)-Ls*u(2))/u(3)
  Flux axe d6 : Fcn  Expr=u(1)-Rs*u(2)-u(3)*u(4)
  Flux axe d7 : Fcn  Expr=-Rr*u(2)+u(1)*u(4)
  Flux axe d8 : Fcn  Expr=-Rr*u(2)-u(1)*u(4)
  Integrator{,1..3} (4 alike) : Integrator
  Mux{1..4} (4 alike) : Mux  Inputs=3
  Mux{5..9} (5 alike) : Mux
  ParkT : Subsystem
      settings: PortSchema="{\"entries\":[{\"content\":{\"sides\":[{\"content\":{\"connectorIds\":[\"In1\"]},\"type\":\"ConnectorPlacement.EquallySpacedRectSide\",\"uuid\":\"228dfcfc-5d6b-4d2b-a954-ee5f3fee8856\"},{\"content\":{\"connectorIds\":[\"Out1\"],\"side\":\"RIGHT\"},\"type\":\"ConnectorPlacement.EquallySpacedRectSide\",\"uuid\":\"1b1b4c30-bceb-4aa5-9a3a-183aa9b64903\"},{\"content\":{\"connectorIds\":[],\"side\":\"TOP\"},\"type\":\"ConnectorPlacement.EquallySpacedRectSide\",\"uuid\":\"f7d3bddd-1df8-4cd8-ab8f-9e5cd0980ffa\"},{\"content\":{\"connectorIds\":[\"In2\"],\"side\":\"BOTTOM\"},\"type\":\"ConnectorPlacement.EquallySpacedRectSide\",\"uuid\":\"ca51e6a4-16df-4fde-8b7d-f74278a3171d\"}]},\"type\":\"ConnectorPlacement.EquallySpacedConnector\",\"uuid\":\"a8efb2f9-24b2-4419-8f97-2809a6aaa24c\"}],\"packageUris\":[\"http://schema.mathworks.com/mf0/Connector/R2020b\"],\"version\":\"1.0\"}"
  Isd : Outport
  Isq : Outport  Port=2
  Torque : Outport  Port=3
  tag scope: Frd=global, Isd=global, Isq=global, Puls_S=global, dFrddt=global
  wires:
  Puls_S/1 -> Add/1, [Puls_S]
  Mux6/1 -> Flux axe d3/1
  [Vsd] -> Mux6/1
  [Isd] -> Mux6/2
  [Puls_S] -> Mux6/3
  [Fsq] -> Mux6/4
  Flux axe d3/1 -> Integrator/1
  Integrator/1 -> [Fsd]
  Mux7/1 -> Flux axe d6/1
  [Vsq] -> Mux7/1
  [Isq] -> Mux7/2
  [Puls_S] -> Mux7/3
  [Fsd] -> Mux7/4
  Flux axe d6/1 -> Integrator1/1
  Integrator1/1 -> [Fsq]
  Mux8/1 -> Flux axe d7/1
  [Ird] -> Mux8/2
  [Puls_S] -> Mux8/3
  [Frq] -> Mux8/4
  Flux axe d7/1 -> [dFrddt], Integrator2/1
  Integrator2/1 -> [Frd]
  Mux9/1 -> Flux axe d8/1
  [Puls_r] -> Mux8/1
  [Irq] -> Mux9/2
  [Puls_S] -> Mux9/3
  [Frd] -> Mux9/4
  Flux axe d8/1 -> Integrator3/1
  Integrator3/1 -> [Frq]
  [Puls_r] -> Mux9/1
  [Frd] -> Mux1/1
  [Fsd] -> Mux1/2
  Mux1/1 -> Flux axe d1/1
  Constant/1 -> Mux1/3
  Flux axe d1/1 -> Isd/1, [Isd]
  [Fsd] -> Mux2/1
  [Frd] -> Mux2/2
  Mux2/1 -> Flux axe d2/1
  Constant1/1 -> Mux2/3
  Flux axe d2/1 -> [Ird]
  [Frq] -> Mux3/1
  [Fsq] -> Mux3/2
  Mux3/1 -> Flux axe d4/1
  Constant2/1 -> Mux3/3
  Flux axe d4/1 -> Isq/1, [Isq]
  [Fsq] -> Mux4/1
  [Frq] -> Mux4/2
  Mux4/1 -> Flux axe d5/1
  Constant3/1 -> Mux4/3
  Flux axe d5/1 -> [Irq]
  Mux5/1 -> Developed Torque/1
  Developed Torque/1 -> Torque/1  "Torque"
  [Isd] -> Mux5/4
  [Fsd] -> Mux5/1
  [Isq] -> Mux5/2
  [Fsq] -> Mux5/3
  Puls_M/1 -> Add/2
  Add/1 -> [Puls_r]
  VABC/1 -> ParkT/1(XABC)
  Demux/2 -> [Vsq]
  Demux/1 -> [Vsd]
  ParkT/1(dq) -> Demux/1
  [thetas] -> ParkT/2(Theta)

== system Copy_of_Clark/IM - Mechanical Behavior ==
  Developed Torque : Inport
  Load Torque : Inport  Port=2
  Add2 : Sum  Inputs=-+
  Transfer Fcn : TransferFcn  Denominator=[J f]
  Speed (rad/s) : Outport
  wires:
  Developed Torque/1 -> Add2/2
  Load Torque/1 -> Add2/1
  Add2/1 -> Transfer Fcn/1
  Transfer Fcn/1 -> Speed (rad/s)/1

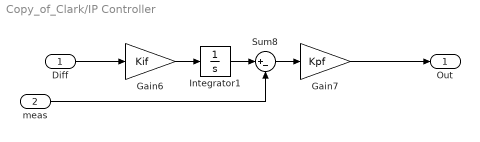
== system Copy_of_Clark/IP Controller ==
  Diff : Inport
  meas : Inport  Port=2
  Gain6 : Gain  Gain=Kif
  Gain7 : Gain  Gain=Kpf
  Integrator1 : Integrator  InitialCondition=0.5/Msr
  Sum8 : Sum  Inputs=|+-
  Out : Outport
  wires:
  Sum8/1 -> Gain7/1
  Integrator1/1 -> Sum8/1
  Gain6/1 -> Integrator1/1
  Diff/1 -> Gain6/1
  meas/1 -> Sum8/2
  Gain7/1 -> Out/1

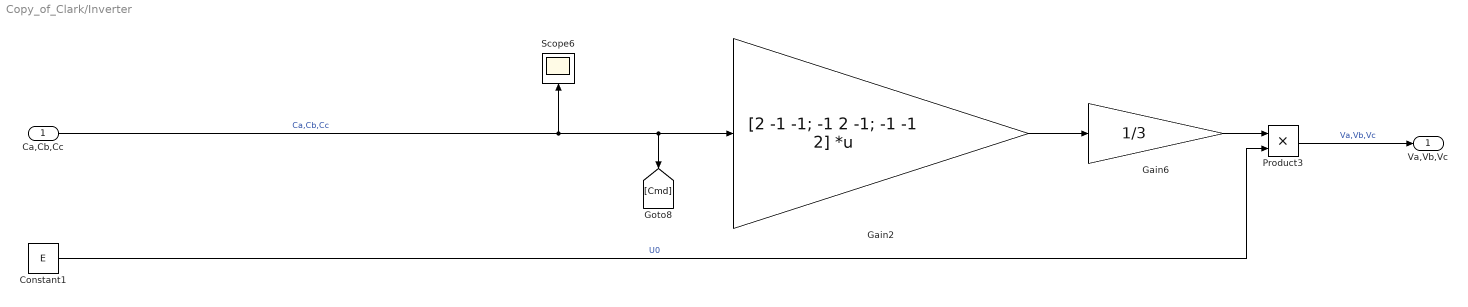
== system Copy_of_Clark/Inverter ==
  Ca,Cb,Cc : Inport
  Constant1 : Constant  Value=E
  Gain2 : Gain  Gain=[2 -1 -1; -1 2 -1; -1 -1 2]  Multiplication=Matrix(K*u)
  Gain6 : Gain  Gain=1/3
  Product3 : Product
  Scope6 : Scope
  Va,Vb,Vc : Outport
  wires:
  Gain2/1 -> Gain6/1
  Product3/1 -> Va,Vb,Vc/1  "Va,Vb,Vc"
  Ca,Cb,Cc/1 -> [Cmd], Gain2/1, Scope6/1  "Ca,Cb,Cc"
  Constant1/1 -> Product3/2  "U0"
  Gain6/1 -> Product3/1

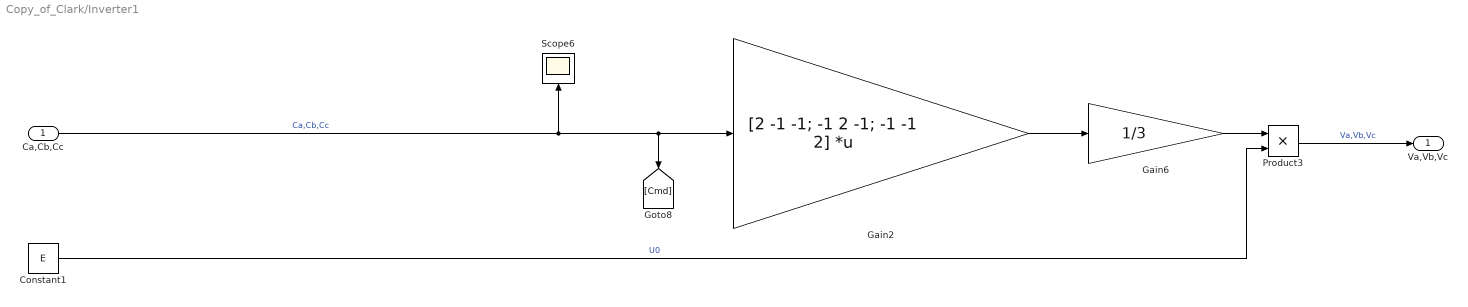
== system Copy_of_Clark/Inverter1 ==
  Ca,Cb,Cc : Inport
  Constant1 : Constant  Value=E
  Gain2 : Gain  Gain=[2 -1 -1; -1 2 -1; -1 -1 2]  Multiplication=Matrix(K*u)
  Gain6 : Gain  Gain=1/3
  Product3 : Product
  Scope6 : Scope
  Va,Vb,Vc : Outport
  wires:
  Gain2/1 -> Gain6/1
  Product3/1 -> Va,Vb,Vc/1  "Va,Vb,Vc"
  Ca,Cb,Cc/1 -> [Cmd], Gain2/1, Scope6/1  "Ca,Cb,Cc"
  Constant1/1 -> Product3/2  "U0"
  Gain6/1 -> Product3/1

== system Copy_of_Clark/Off time per sector calculator ==
  taoff,tboff,tcoff : Inport
  sector : Inport  Port=2
  Off time per sector calculator : MATLAB Function  TreatAsAtomicUnit=on
  Tmat : Outport
  wires:
  Off time per sector calculator/1(Tmat) -> Tmat/1
  sector/1 -> Off time per sector calculator/2(sector)
  taoff,tboff,tcoff/1 -> Off time per sector calculator/1(toff)

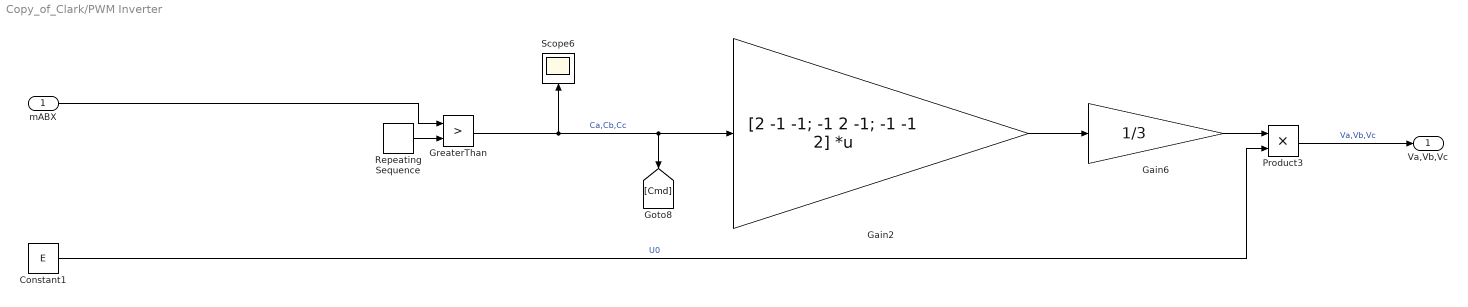
== system Copy_of_Clark/PWM Inverter ==
  mABX : Inport
  Constant1 : Constant  Value=E
  Gain2 : Gain  Gain=[2 -1 -1; -1 2 -1; -1 -1 2]  Multiplication=Matrix(K*u)
  Gain6 : Gain  Gain=1/3
  GreaterThan : RelationalOperator  Operator=>  OutDataTypeStr=boolean  RndMeth=Simplest  InputSameDT=off
  Product3 : Product
  Repeating Sequence : simulink/Sources/Repeating Sequence  rep_seq_t=[0 Ts]  rep_seq_y=[-1 1]
  Scope6 : Scope
  Va,Vb,Vc : Outport
  wires:
  Gain2/1 -> Gain6/1
  Product3/1 -> Va,Vb,Vc/1  "Va,Vb,Vc"
  mABX/1 -> GreaterThan/1
  GreaterThan/1 -> [Cmd], Gain2/1, Scope6/1  "Ca,Cb,Cc"
  Repeating Sequence/1 -> GreaterThan/2
  Constant1/1 -> Product3/2  "U0"
  Gain6/1 -> Product3/1

== system Copy_of_Clark/ParkT-2 ==
  dq : Inport
  Theta : Inport  Port=2
  MATLAB Function : MATLAB Function  TreatAsAtomicUnit=on
  XABC : Outport
  wires:
  Theta/1 -> MATLAB Function/2(th)
  dq/1 -> MATLAB Function/1(dq)
  MATLAB Function/1(XABC) -> XABC/1

== system Copy_of_Clark/ParkT-3 ==
  dq : Inport
  Theta : Inport  Port=2
  MATLAB Function : MATLAB Function  TreatAsAtomicUnit=on
  XABC : Outport
  wires:
  MATLAB Function/1(XABC) -> XABC/1
  dq/1 -> MATLAB Function/1(dq)
  Theta/1 -> MATLAB Function/2(th)

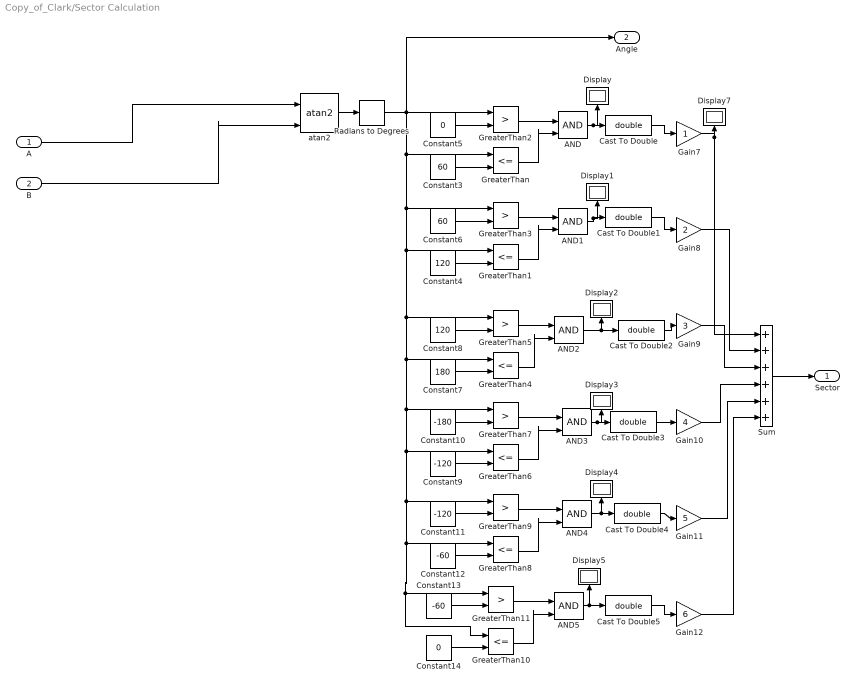
== system Copy_of_Clark/Sector Calculation ==
  A : Inport
  B : Inport  Port=2
  AND{,1..5} (6 alike) : Logic  IconShape=distinctive  AllPortsSameDT=off  OutDataTypeStr=boolean
  Cast To Double{,1..5} (6 alike) : DataTypeConversion  OutDataTypeStr=double  SaturateOnIntegerOverflow=off  RndMeth=Floor
  Constant10 : Constant  Value=-180
  Constant11 : Constant  Value=-120
  Constant12 : Constant  Value=-60
  Constant13 : Constant  Value=-60
  Constant14 : Constant  Value=0
  Constant3 : Constant  Value=60
  Constant4 : Constant  Value=120
  Constant5 : Constant  Value=0
  Constant6 : Constant  Value=60
  Constant7 : Constant  Value=180
  Constant8 : Constant  Value=120
  Constant9 : Constant  Value=-120
  Display{,1..5,7} (7 alike) : Display
  Gain10 : Gain  Gain=4
  Gain11 : Gain  Gain=5
  Gain12 : Gain  Gain=6
  Gain7 : Gain
  Gain8 : Gain  Gain=2
  Gain9 : Gain  Gain=3
  GreaterThan{,1,4,6,8,10} (6 alike) : RelationalOperator  Operator=<=  OutDataTypeStr=boolean  RndMeth=Simplest  InputSameDT=off
  GreaterThan{2..3,5,7,9,11} (6 alike) : RelationalOperator  Operator=>  OutDataTypeStr=boolean  RndMeth=Simplest  InputSameDT=off
  Radians to Degrees : simulink_extras/Transformations/Radians to Degrees
  Sum : Sum  Inputs=++++++
  atan2 : mcbcontrolslib/atan2  outputUnit=Radians
      settings: LibrarySourceBlock=mcblib/Controls/Math Transforms/atan2
  Sector : Outport
  Angle : Outport  Port=2
  wires:
  AND1/1 -> Display1/1, Cast To Double1/1
  GreaterThan5/1 -> AND2/1
  GreaterThan10/1 -> AND5/2
  Radians to Degrees/1 -> Angle/1, GreaterThan10/1, GreaterThan11/1, GreaterThan8/1, GreaterThan9/1, GreaterThan6/1, GreaterThan7/1, GreaterThan4/1, GreaterThan5/1, GreaterThan1/1, GreaterThan3/1, GreaterThan/1, GreaterThan2/1
  Constant4/1 -> GreaterThan1/2
  GreaterThan3/1 -> AND1/1
  Constant14/1 -> GreaterThan10/2
  GreaterThan1/1 -> AND1/2
  GreaterThan8/1 -> AND4/2
  Gain8/1 -> Sum/2
  Constant13/1 -> GreaterThan11/2
  Gain12/1 -> Sum/6
  GreaterThan4/1 -> AND2/2
  AND2/1 -> Display2/1, Cast To Double2/1
  Gain9/1 -> Sum/3
  GreaterThan/1 -> AND/2
  GreaterThan6/1 -> AND3/2
  Constant8/1 -> GreaterThan5/2
  AND5/1 -> Display5/1, Cast To Double5/1
  AND/1 -> Display/1, Cast To Double/1
  AND4/1 -> Display4/1, Cast To Double4/1
  Constant7/1 -> GreaterThan4/2
  Constant10/1 -> GreaterThan7/2
  Constant12/1 -> GreaterThan8/2
  Constant5/1 -> GreaterThan2/2
  Constant11/1 -> GreaterThan9/2
  Cast To Double4/1 -> Gain11/1
  GreaterThan9/1 -> AND4/1
  Gain11/1 -> Sum/5
  Gain10/1 -> Sum/4
  GreaterThan11/1 -> AND5/1
  Cast To Double/1 -> Gain7/1
  Constant9/1 -> GreaterThan6/2
  GreaterThan2/1 -> AND/1
  Cast To Double3/1 -> Gain10/1
  Constant3/1 -> GreaterThan/2
  Cast To Double2/1 -> Gain9/1
  GreaterThan7/1 -> AND3/1
  Gain7/1 -> Sum/1, Display7/1
  Constant6/1 -> GreaterThan3/2
  Cast To Double5/1 -> Gain12/1
  Cast To Double1/1 -> Gain8/1
  A/1 -> atan2/1
  B/1 -> atan2/2
  Sum/1 -> Sector/1
  atan2/1 -> Radians to Degrees/1
  AND3/1 -> Display3/1, Cast To Double3/1

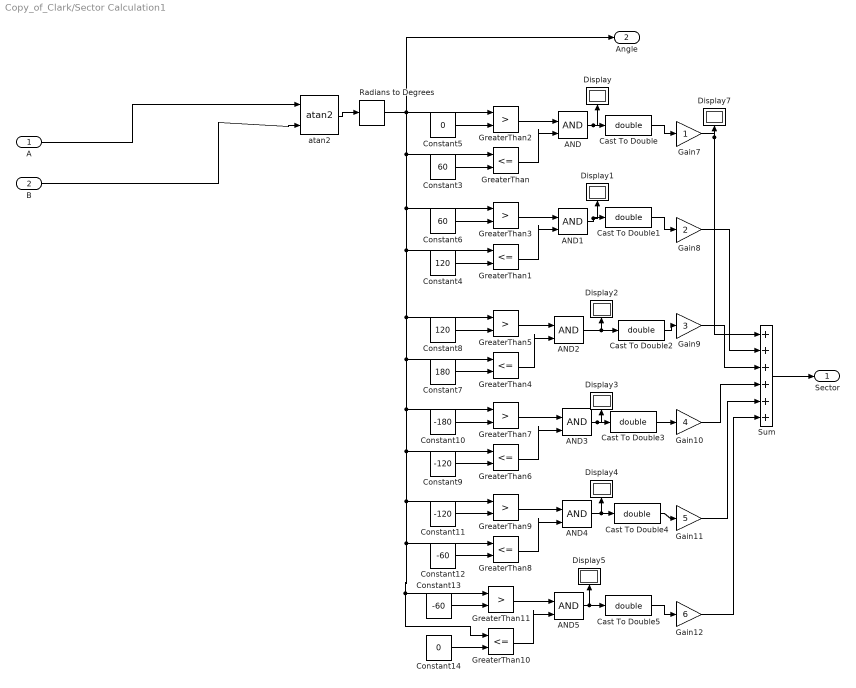
== system Copy_of_Clark/Sector Calculation1 ==
  A : Inport
  B : Inport  Port=2
  AND{,1..5} (6 alike) : Logic  IconShape=distinctive  AllPortsSameDT=off  OutDataTypeStr=boolean
  Cast To Double{,1..5} (6 alike) : DataTypeConversion  OutDataTypeStr=double  SaturateOnIntegerOverflow=off  RndMeth=Floor
  Constant10 : Constant  Value=-180
  Constant11 : Constant  Value=-120
  Constant12 : Constant  Value=-60
  Constant13 : Constant  Value=-60
  Constant14 : Constant  Value=0
  Constant3 : Constant  Value=60
  Constant4 : Constant  Value=120
  Constant5 : Constant  Value=0
  Constant6 : Constant  Value=60
  Constant7 : Constant  Value=180
  Constant8 : Constant  Value=120
  Constant9 : Constant  Value=-120
  Display{,1..5,7} (7 alike) : Display
  Gain10 : Gain  Gain=4
  Gain11 : Gain  Gain=5
  Gain12 : Gain  Gain=6
  Gain7 : Gain
  Gain8 : Gain  Gain=2
  Gain9 : Gain  Gain=3
  GreaterThan{,1,4,6,8,10} (6 alike) : RelationalOperator  Operator=<=  OutDataTypeStr=boolean  RndMeth=Simplest  InputSameDT=off
  GreaterThan{2..3,5,7,9,11} (6 alike) : RelationalOperator  Operator=>  OutDataTypeStr=boolean  RndMeth=Simplest  InputSameDT=off
  Radians to Degrees : simulink_extras/Transformations/Radians to Degrees
  Sum : Sum  Inputs=++++++
  atan2 : mcbcontrolslib/atan2  outputUnit=Radians
      settings: LibrarySourceBlock=mcblib/Controls/Math Transforms/atan2
  Sector : Outport
  Angle : Outport  Port=2
  wires:
  AND3/1 -> Cast To Double3/1, Display3/1
  atan2/1 -> Radians to Degrees/1
  Sum/1 -> Sector/1
  B/1 -> atan2/2
  A/1 -> atan2/1
  Cast To Double1/1 -> Gain8/1
  Cast To Double5/1 -> Gain12/1
  Constant6/1 -> GreaterThan3/2
  Gain7/1 -> Display7/1, Sum/1
  GreaterThan7/1 -> AND3/1
  Cast To Double2/1 -> Gain9/1
  Constant3/1 -> GreaterThan/2
  Cast To Double3/1 -> Gain10/1
  GreaterThan2/1 -> AND/1
  Constant9/1 -> GreaterThan6/2
  Cast To Double/1 -> Gain7/1
  GreaterThan11/1 -> AND5/1
  Gain10/1 -> Sum/4
  Gain11/1 -> Sum/5
  GreaterThan9/1 -> AND4/1
  Cast To Double4/1 -> Gain11/1
  Constant11/1 -> GreaterThan9/2
  Constant5/1 -> GreaterThan2/2
  Constant12/1 -> GreaterThan8/2
  Constant10/1 -> GreaterThan7/2
  Constant7/1 -> GreaterThan4/2
  AND4/1 -> Cast To Double4/1, Display4/1
  AND/1 -> Cast To Double/1, Display/1
  AND5/1 -> Cast To Double5/1, Display5/1
  Constant8/1 -> GreaterThan5/2
  GreaterThan6/1 -> AND3/2
  GreaterThan/1 -> AND/2
  Gain9/1 -> Sum/3
  AND2/1 -> Cast To Double2/1, Display2/1
  GreaterThan4/1 -> AND2/2
  Gain12/1 -> Sum/6
  Constant13/1 -> GreaterThan11/2
  Gain8/1 -> Sum/2
  GreaterThan8/1 -> AND4/2
  GreaterThan1/1 -> AND1/2
  Constant14/1 -> GreaterThan10/2
  GreaterThan3/1 -> AND1/1
  Constant4/1 -> GreaterThan1/2
  Radians to Degrees/1 -> GreaterThan2/1, GreaterThan/1, GreaterThan3/1, GreaterThan1/1, GreaterThan5/1, GreaterThan4/1, GreaterThan7/1, GreaterThan6/1, GreaterThan9/1, GreaterThan8/1, GreaterThan11/1, GreaterThan10/1, Angle/1
  GreaterThan10/1 -> AND5/2
  GreaterThan5/1 -> AND2/1
  AND1/1 -> Cast To Double1/1, Display1/1

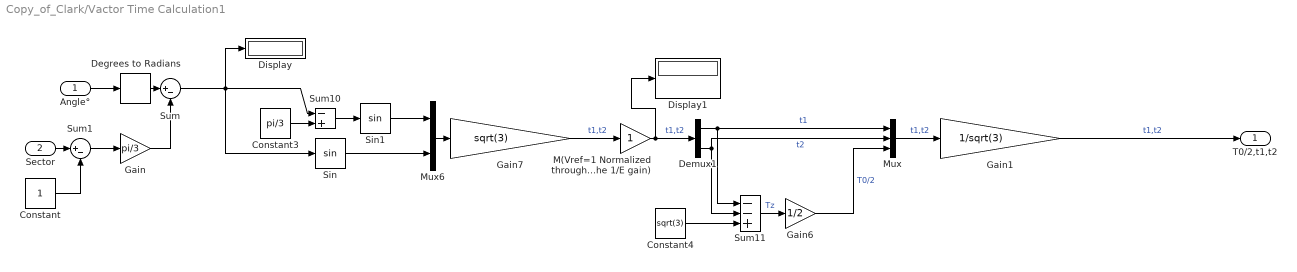
== system Copy_of_Clark/Vactor Time Calculation1 ==
  Angle° : Inport
  Sector : Inport  Port=2
  Constant : Constant
  Constant3 : Constant  Value=pi/3
  Constant4 : Constant  Value=sqrt(3)
  Degrees to Radians : simulink_extras/Transformations/Degrees to Radians
  Demux1 : Demux  Outputs=2
  Display : Display
  Display1 : Display
  Gain : Gain  Gain=pi/3
  Gain1 : Gain  Gain=1/sqrt(3)
  Gain6 : Gain  Gain=1/2
  Gain7 : Gain  Gain=sqrt(3)
  M(Vref=1 Normalized through the 1/E gain) : Gain
  Mux : Mux  Inputs=3
  Mux6 : Mux  Inputs=2
  Sin : Trigonometry
  Sin1 : Trigonometry
  Sum : Sum  Inputs=|+-
  Sum1 : Sum  Inputs=|+-
  Sum10 : Sum  Inputs=-+
  Sum11 : Sum  Inputs=--+
  T0/2,t1,t2 : Outport
  wires:
  Constant4/1 -> Sum11/3
  Sum11/1 -> Gain6/1  "Tz"
  Demux1/1 -> Mux/1, Sum11/1  "t1"
  Demux1/2 -> Mux/2, Sum11/2  "t2"
  Mux6/1 -> Gain7/1
  M(Vref=1 Normalized through the 1/E gain)/1 -> Display1/1, Demux1/1  "t1,t2"
  Gain6/1 -> Mux/3  "T0/2"
  Angle°/1 -> Degrees to Radians/1
  Sin/1 -> Mux6/2
  Sin1/1 -> Mux6/1
  Constant3/1 -> Sum10/2
  Sum10/1 -> Sin1/1
  Sum/1 -> Sin/1, Display/1, Sum10/1
  Gain7/1 -> M(Vref=1 Normalized through the 1/E gain)/1  "t1,t2"
  Mux/1 -> Gain1/1  "t1,t2"
  Gain1/1 -> T0/2,t1,t2/1  "t1,t2"
  Degrees to Radians/1 -> Sum/1
  Gain/1 -> Sum/2
  Sector/1 -> Sum1/1
  Constant/1 -> Sum1/2
  Sum1/1 -> Gain/1

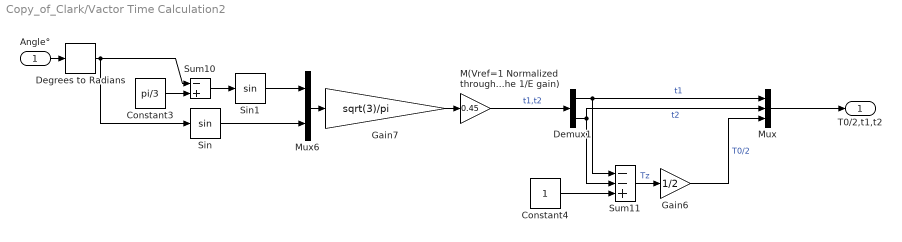
== system Copy_of_Clark/Vactor Time Calculation2 ==
  Angle° : Inport
  Constant3 : Constant  Value=pi/3
  Constant4 : Constant
  Degrees to Radians : simulink_extras/Transformations/Degrees to Radians
  Demux1 : Demux  Outputs=2
  Gain6 : Gain  Gain=1/2
  Gain7 : Gain  Gain=sqrt(3)/pi
  M(Vref=1 Normalized through the 1/E gain) : Gain  Gain=0.45
  Mux : Mux  Inputs=3
  Mux6 : Mux  Inputs=2
  Sin : Trigonometry
  Sin1 : Trigonometry
  Sum10 : Sum  Inputs=-+
  Sum11 : Sum  Inputs=--+
  T0/2,t1,t2 : Outport
  wires:
  Constant4/1 -> Sum11/3
  Sum11/1 -> Gain6/1  "Tz"
  Demux1/1 -> Mux/1, Sum11/1  "t1"
  Demux1/2 -> Mux/2, Sum11/2  "t2"
  Gain7/1 -> M(Vref=1 Normalized through the 1/E gain)/1
  Mux6/1 -> Gain7/1
  M(Vref=1 Normalized through the 1/E gain)/1 -> Demux1/1  "t1,t2"
  Gain6/1 -> Mux/3  "T0/2"
  Mux/1 -> T0/2,t1,t2/1
  Angle°/1 -> Degrees to Radians/1
  Sin/1 -> Mux6/2
  Sin1/1 -> Mux6/1
  Constant3/1 -> Sum10/2
  Sum10/1 -> Sin1/1
  Degrees to Radians/1 -> Sin/1, Sum10/1

== system Copy_of_Clark/IM - Electric Behavior/ParkT ==
  XABC : Inport
  Theta : Inport  Port=2
  MATLAB Function1 : MATLAB Function  TreatAsAtomicUnit=on
  dq : Outport
  wires:
  Theta/1 -> MATLAB Function1/2(th)
  MATLAB Function1/1(dq) -> dq/1
  XABC/1 -> MATLAB Function1/1(x)

== matlab function Copy_of_Clark/ClarkT/MATLAB Function1 ==
  data: x input; alpha output; beta output
function [alpha,beta] = Clark(x)
P=(2/3)*[ cos(0) cos(0-2*pi/3) cos(0+2*pi/3);
         -sin(0) -sin(0-2*pi/3) -sin(0+2*pi/3)  ];
prod=P*x;
alpha=prod(1);
beta=prod(2);

== matlab function Copy_of_Clark/ClarkT-1/MATLAB Function ==
  data: alpha input; beta input; XABC output
function XABC= Clarkinv(alpha,beta)

parkinv = [ cos(0),           -sin(0); 
          cos(0-2*pi/3), -sin(0-2*pi/3); 
          cos(0+2*pi/3), -sin(0+2*pi/3)];

XABC = parkinv * [alpha;beta];

% x1=temp(1);
% x2=temp(2);
% x3=temp(3);

== matlab function Copy_of_Clark/ClarkT-2/MATLAB Function ==
  data: alpha input; beta input; XABC output
function XABC= Clarkinv(alpha,beta)

parkinv = [ cos(0),           -sin(0); 
          cos(0-2*pi/3), -sin(0-2*pi/3); 
          cos(0+2*pi/3), -sin(0+2*pi/3)];

XABC = parkinv * [alpha;beta];

% x1=temp(1);
% x2=temp(2);
% x3=temp(3);

== matlab function Copy_of_Clark/ClarkT1/MATLAB Function1 ==
  data: x input; alpha output; beta output
function [alpha,beta] = Clark(x)
P=(2/3)*[ cos(0) cos(0-2*pi/3) cos(0+2*pi/3);
         -sin(0) -sin(0-2*pi/3) -sin(0+2*pi/3)  ];
prod=P*x;
alpha=prod(1);
beta=prod(2);

== matlab function Copy_of_Clark/IM - Electric Behavior/ParkT/MATLAB Function1 ==
  data: x input; dq output; th input
function dq = Park(x,th)
% vd=(2/3)*(u1*cos(th)+u2*cos(th-2*pi/3)+u3*cos(th+2*pi/3));
% vq=(2/3)*(-u1*sin(th)-u2*sin(th-2*pi/3)-u3*sin(th+2*pi/3));
P=(2/3)*[ cos(th) cos(th-2*pi/3) cos(th+2*pi/3);
         -sin(th) -sin(th-2*pi/3) -sin(th+2*pi/3)  ];
dq=P*x;
% xd=prod(1);
% xq=prod(2);

== matlab function Copy_of_Clark/ParkT-2/MATLAB Function ==
  data: dq input; XABC output; th input
function XABC= Parkinv(dq,th)

parkinv = [ cos(th),           -sin(th); 
          cos(th-2*pi/3), -sin(th-2*pi/3); 
          cos(th+2*pi/3), -sin(th+2*pi/3)];

XABC = parkinv * [dq];

% x1=temp(1);
% x2=temp(2);
% x3=temp(3);

== matlab function Copy_of_Clark/ParkT-3/MATLAB Function ==
  data: dq input; XABC output; th input
function XABC= Parkinv(dq,th)

parkinv = [ cos(th),           -sin(th); 
          cos(th-2*pi/3), -sin(th-2*pi/3); 
          cos(th+2*pi/3), -sin(th+2*pi/3)];

XABC = parkinv * [dq];

% x1=temp(1);
% x2=temp(2);
% x3=temp(3);

== matlab function Copy_of_Clark/ClarkT2/MATLAB Function1 ==
  data: x input; alpha output; beta output
function [alpha,beta] = Clark(x)
P=(2/3)*[ cos(0) cos(0-2*pi/3) cos(0+2*pi/3);
         -sin(0) -sin(0-2*pi/3) -sin(0+2*pi/3)  ];
prod=P*x;
alpha=prod(1);
beta=prod(2);

== matlab function Copy_of_Clark/Off time per sector calculator/Off time per sector calculator ==
  data: toff input; Tmat output; sector input
function Tmat = Sectortime(toff,sector)


switch sector
    case 1
        Tmat=toff(1:3);
    case 2
        Tmat=toff(4:6);
    case 3
        Tmat=toff(7:9);
    case 4
        Tmat=toff(10:12);
    case 5
        Tmat=toff(13:15);
    case 6
        Tmat=toff(16:18);
    otherwise
        Tmat=[nan;nan;nan];
end
